simulink model "Offline_SCGAnalysis_3DModCalculator"  (R2019a)
settings: Solver=FixedStepDiscrete  StartTime=0.0  StopTime=param_sim_time  FixedStep=1/fs  MaxStep=1/fs  RelTol=1e-3
settings Model: PacingRate=100  Creator=rcord  LastModifiedBy=rcord
settings SolverCC: ZeroCrossControl=DisableAll
settings DataIOCC: ExternalInput=[t, signals.scg.preprocessing_x, signals.scg.preprocessing_y, signals.scg.preprocessing_z]  LoadExternalInput=on  SignalLogging=off  DSMLogging=off  SaveTime=off  ReturnWorkspaceOutputs=off  TimeSaveName=t_preprocessing  OutputSaveName=out_preprocessing  LoggingIntervals=[-inf,inf]

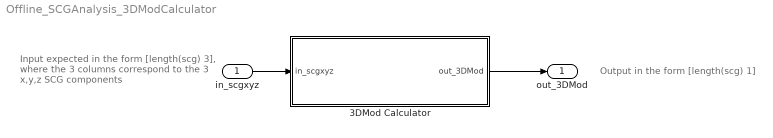
== system Offline_SCGAnalysis_3DModCalculator ==
  note: Output in the form [length(scg) 1]
  note: Input expected in the form [length(scg) 3],
      | where the 3 columns correspond to the
      | 3 x,y,z SCG components
  in_scgxyz : Inport
  3DMod Calculator : Subsystem
  out_3DMod : Outport
  wires:
  in_scgxyz/1 -> 3DMod Calculator/1(in_scgxyz)
  3DMod Calculator/1(out_3DMod) -> out_3DMod/1

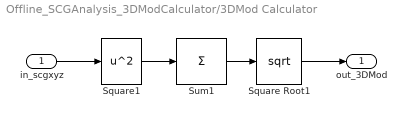
== system Offline_SCGAnalysis_3DModCalculator/3DMod Calculator ==
  in_scgxyz : Inport
  Square Root1 : Sqrt  SaturateOnIntegerOverflow=on
  Square1 : Math  Operator=square  SaturateOnIntegerOverflow=on
  Sum1 : Sum  Inputs=+  CollapseMode=Specified dimension  CollapseDim=2
  out_3DMod : Outport
  wires:
  Square1/1 -> Sum1/1
  Sum1/1 -> Square Root1/1
  in_scgxyz/1 -> Square1/1
  Square Root1/1 -> out_3DMod/1
